simulink model "plant_model"  (R2018b)
settings: Solver=VariableStepAuto  StartTime=0.0  StopTime=10.0  RelTol=1e-3
values from neighbouring files (symbols this model uses):
  alpha_i = 5/37.5    (= 0.133333333333)    [drv_sen_sim.m]    (also in plant_model_sim.m)
  alpha_T = 1.5/1000    (= 0.0015)    [plant_model_sim.m]    (also in sensor_sim.m)
  D = 6.0e-5    (= 6e-05)    [motor_sim.m]    (also in plant_model_sim.m)
  Ji = 1.3e-3    (= 0.0013)    [motor_sim.m]    (also in plant_model_sim.m)
  Jm = 0.11e-3    (= 0.00011)    [motor_sim.m]    (also in plant_model_sim.m)
  Ke = 7.16e-2    (= 0.0716)    [motor_sim.m]    (also in plant_model_sim.m)
  Kt = 7.2e-2    (= 0.072)    [motor_sim.m]    (also in plant_model_sim.m)
  L = 0.2    [motor_sim.m]    (also in plant_model_sim.m)
  R = 5.7    [motor_sim.m]    (also in plant_model_sim.m)
  u_M_d = 10    [drv_sen_sim.m]    (also in plant_model_sim.m)
  Vin = 24    [drv_sen_sim.m]    (also in plant_model_sim.m)
settings Model: Creator=nharada  LastModifiedBy=nharada

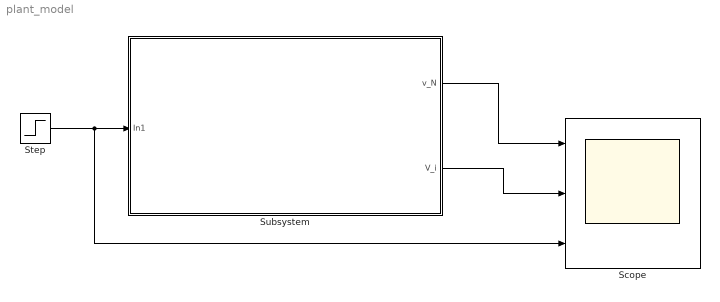
== system plant_model ==
  Scope : Scope  NumInputPorts=3
  Step : Step  After=u_M_d  SampleTime=0
  Subsystem : Subsystem
  wires:
  Subsystem/1("v_N ") -> Scope/1
  Subsystem/2(V_i) -> Scope/2
  Step/1 -> Scope/3, Subsystem/1(In1)

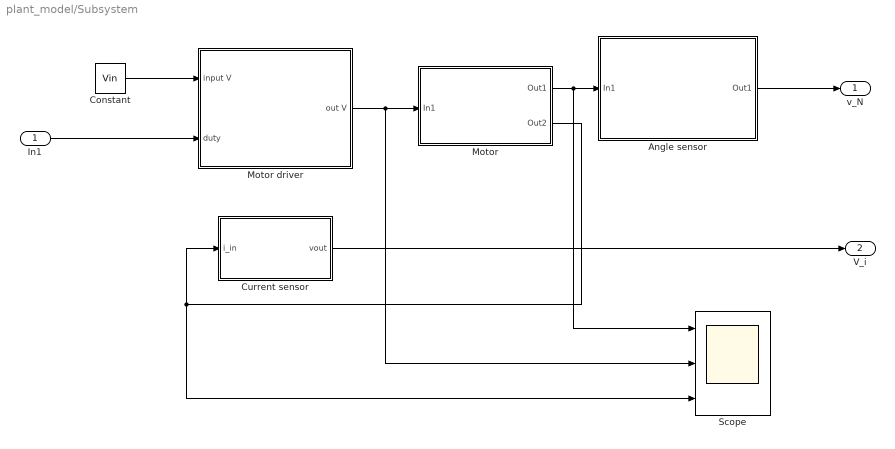
== system plant_model/Subsystem ==
  In1 : Inport
  Angle sensor : Subsystem
  Constant : Constant  Value=Vin
  Current sensor : Subsystem
  Motor : Subsystem
  Motor driver : Subsystem
  Scope : Scope  NumInputPorts=3
  "v_N " : Outport
  V_i : Outport  Port=2
  wires:
  Current sensor/1(vout) -> V_i/1
  Constant/1 -> Motor driver/1(input V)
  Motor driver/1(out V) -> Scope/2, Motor/1(In1)
  Motor/2(Out2) -> Current sensor/1(i_in), Scope/3
  Motor/1(Out1) -> Scope/1, Angle sensor/1(In1)
  In1/1 -> Motor driver/2(duty)
  Angle sensor/1(Out1) -> "v_N "/1

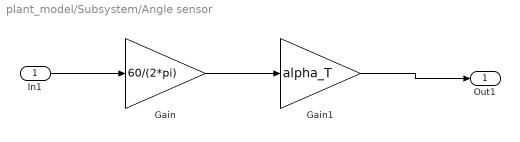
== system plant_model/Subsystem/Angle sensor ==
  In1 : Inport
  Gain : Gain  Gain=60/(2*pi)
  Gain1 : Gain  Gain=alpha_T
  Out1 : Outport
  wires:
  In1/1 -> Gain/1
  Gain/1 -> Gain1/1
  Gain1/1 -> Out1/1

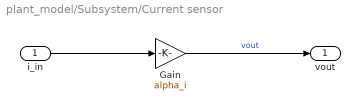
== system plant_model/Subsystem/Current sensor ==
  i_in : Inport
  Gain : Gain  Gain=alpha_i
  vout : Outport
  wires:
  Gain/1 -> vout/1  "vout"
  i_in/1 -> Gain/1

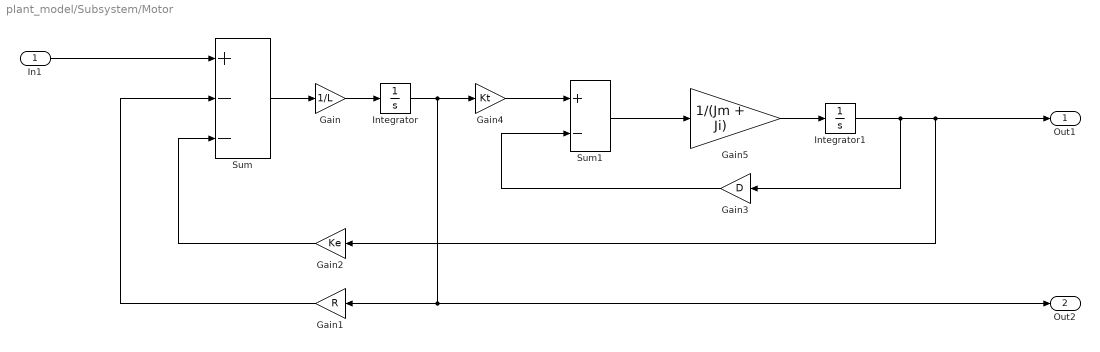
== system plant_model/Subsystem/Motor ==
  In1 : Inport
  Gain : Gain  Gain=1/L
  Gain1 : Gain  Gain=R
  Gain2 : Gain  Gain=Ke
  Gain3 : Gain  Gain=D
  Gain4 : Gain  Gain=Kt
  Gain5 : Gain  Gain=1/(Jm + Ji)
  Integrator : Integrator
  Integrator1 : Integrator
  Sum : Sum  Inputs=+--
  Sum1 : Sum  Inputs=+-
  Out1 : Outport
  Out2 : Outport  Port=2
  wires:
  Gain1/1 -> Sum/2
  Sum/1 -> Gain/1
  Gain3/1 -> Sum1/2
  Gain2/1 -> Sum/3
  Gain/1 -> Integrator/1
  Integrator1/1 -> Gain3/1, Out1/1, Gain2/1
  Integrator/1 -> Gain4/1, Out2/1, Gain1/1
  Sum1/1 -> Gain5/1
  Gain5/1 -> Integrator1/1
  Gain4/1 -> Sum1/1
  In1/1 -> Sum/1

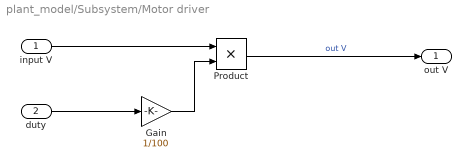
== system plant_model/Subsystem/Motor driver ==
  input V : Inport
  duty : Inport  Port=2
  Gain : Gain  Gain=1/100
  Product : Product
  out V : Outport
  wires:
  Gain/1 -> Product/2
  input V/1 -> Product/1
  Product/1 -> out V/1  "out V"
  duty/1 -> Gain/1
